simulink model "trimming_find_initial_value"  (R2022a)
settings: Solver=VariableStepAuto  StartTime=0.0  StopTime=0.1  RelTol=1e-3
values from neighbouring files (symbols this model uses):
  h = xMax-xMin    [LP_BasicSolution.m]    (also in LP_def.m = [uMax-up; LP_lift.m = [uMax-up; LP_sig.m = [uMax-up; LP_thrust.m = [uMax-up)
  m = m1-1    [CGIwrap.m]    (also in DAISY_CHAINING.m; DA_Allocation.m; LP_BasicSolution.m; LP_def.m)
undefined symbols (not defined in the file or in its folder): ft, kg, km, s, slug
libraries: aerolibconvert2 x12, sharedtransform x2, aerolibatmos2 x1
settings Model: Creator=user
settings SolverCC: AlgebraicLoopSolver=TrustRegion
settings DebuggingCC: UnconnectedInputMsg=warning  UnconnectedOutputMsg=warning  UnconnectedLineMsg=warning  SFMachineParentedDataDiag=warning

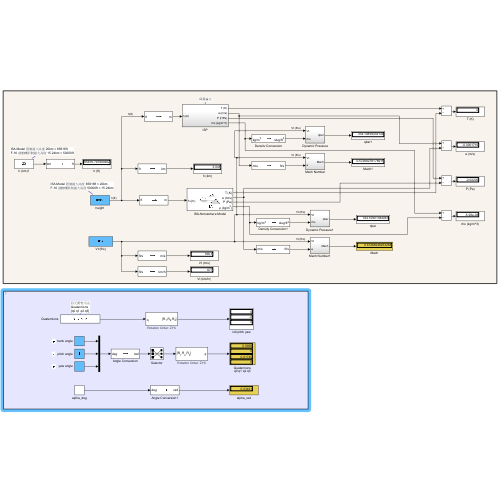
[thumbnail: Simulink's stored preview of the top-level diagram]
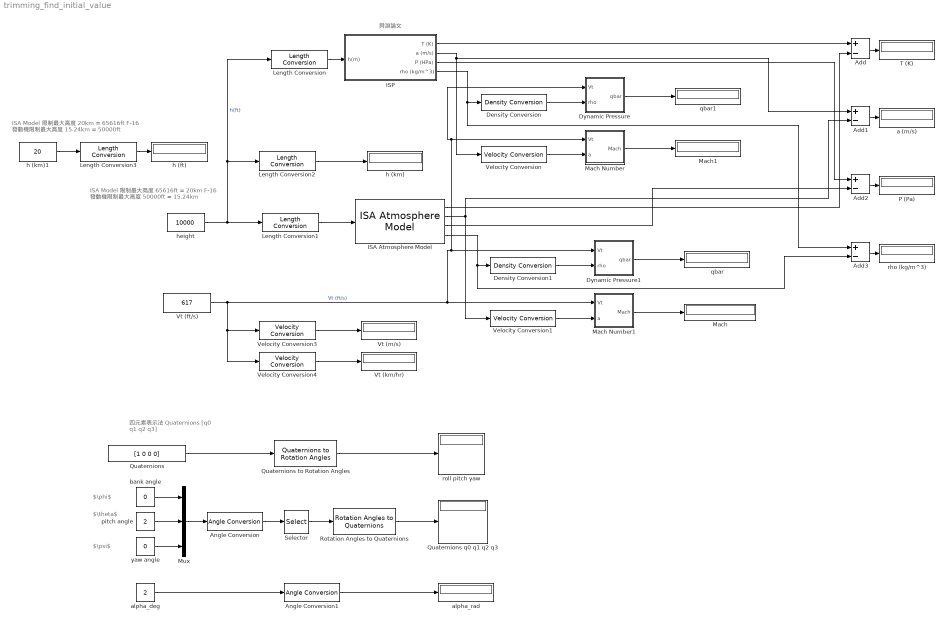
== system trimming_find_initial_value ==
  note: $\phi$
  note: 舜淵論文
  note: ISA Model 限制最大高度 65616ft = 20km
      | F-16 發動機限制最大高度 50000ft = 15.24km
  note: ISA Model 限制最大高度 20km = 65616ft
      | F-16 發動機限制最大高度 15.24km = 50000ft
  note: 四元素表示法
      | Quaternions
      | [q0 q1 q2 q3]
  note: $\theta$
  note: $\psi$
  Add{,1..3} (4 alike) : Sum  Inputs=+-
  Angle Conversion : aerolibconvert2/Angle Conversion  IU=deg  OU=rad
  Angle Conversion1 : aerolibconvert2/Angle Conversion  IU=deg  OU=rad
  Density Conversion : aerolibconvert2/Density Conversion  IU=kg/m^3  OU=slug/ft^3
      settings: SourceProductBaseCode=AE
  Density Conversion1 : aerolibconvert2/Density Conversion  IU=kg/m^3  OU=slug/ft^3
      settings: SourceProductBaseCode=AE
  Dynamic Pressure : Subsystem
  Dynamic Pressure1 : Subsystem
  ISA Atmosphere Model : aerolibatmos2/ISA Atmosphere Model  custom=off  g=9.80665  gamma=1.4  R=287.0531  L=0.0065  h_trop=11000  h_strat=20000  rho0=1.225  P0=101325  T0=288.15  h0=0
  "ISP " : Subsystem
  Length Conversion : aerolibconvert2/Length Conversion  IU=ft  OU=m
  Length Conversion1 : aerolibconvert2/Length Conversion  IU=ft  OU=m
  Length Conversion2 : aerolibconvert2/Length Conversion  IU=ft  OU=km
  Length Conversion3 : aerolibconvert2/Length Conversion  IU=km  OU=ft
  Mach : Display
  Mach Number : Subsystem
  Mach Number1 : Subsystem
  Mach1 : Display
  Mux : Mux  Inputs=3
  P (Pa) : Display
  Quaternions : Constant  Value=[1 0 0 0]
  Quaternions q0 q1 q2 q3 : Display
  Quaternions to Rotation Angles : sharedtransform/Quaternions to Rotation Angles  rotationOrder=ZYX  aMode=aMode
      settings: SourceProductBaseCode=AE,PW,DR,MT,VE
  Rotation Angles to Quaternions : sharedtransform/Rotation Angles to Quaternions  rotationOrder=ZYX  aMode=aMode
      settings: SourceProductBaseCode=AE,PW,DR,MT,VE
  Selector : Selector  InputPortWidth=3  IndexOptions=Index vector (dialog)  Indices=[3 2 1]  OutputSizes=1
  T (K) : Display
  Velocity Conversion : aerolibconvert2/Velocity Conversion  IU=m/s  OU=ft/s
  Velocity Conversion1 : aerolibconvert2/Velocity Conversion  IU=m/s  OU=ft/s
  Velocity Conversion3 : aerolibconvert2/Velocity Conversion  IU=ft/s  OU=m/s
  Velocity Conversion4 : aerolibconvert2/Velocity Conversion  IU=ft/s  OU=km/h
  Vt (ft/s) : Constant  Value=617
  Vt (km/hr) : Display
  Vt (m/s) : Display
  a (m/s) : Display
  alpha_deg : Constant  Value=2
  alpha_rad : Display
  bank angle : Constant  Value=0
  h (ft) : Display
  h (km) : Display
  h (km)1 : Constant  Value=20
  height : Constant  Value=10000
  pitch angle : Constant  Value=2
  qbar : Display
  qbar1 : Display
  rho (kg/m^3) : Display
  roll pitch yaw : Display
  yaw angle : Constant  Value=0
  wires:
  "ISP "/4(rho (kg/m^3)) -> Add3/1, Density Conversion/1
  "ISP "/3(P (HPa)) -> Add2/1
  "ISP "/2(a (m/s)) -> Add1/1, Velocity Conversion/1
  Dynamic Pressure/1(qbar) -> qbar1/1
  Mach Number/1(Mach) -> Mach1/1
  Density Conversion/1 -> Dynamic Pressure/2(rho)
  height/1 -> Length Conversion2/1, Length Conversion/1, Length Conversion1/1  "h(ft)"
  Length Conversion/1 -> "ISP "/1(h(m))
  Vt (ft/s)/1 -> Velocity Conversion4/1, Velocity Conversion3/1, Dynamic Pressure/1(Vt), Mach Number/1(Vt), Dynamic Pressure1/1(Vt), Mach Number1/1(Vt)  "Vt (ft/s)"
  Velocity Conversion/1 -> Mach Number/2(a)
  "ISP "/1(T (K)) -> Add/1
  Velocity Conversion1/1 -> Mach Number1/2(a)
  Length Conversion1/1 -> ISA Atmosphere Model/1
  ISA Atmosphere Model/3 -> Add2/2
  ISA Atmosphere Model/4 -> Add3/2, Density Conversion1/1
  Density Conversion1/1 -> Dynamic Pressure1/2(rho)
  ISA Atmosphere Model/1 -> Add/2
  ISA Atmosphere Model/2 -> Add1/2, Velocity Conversion1/1
  Dynamic Pressure1/1(qbar) -> qbar/1
  Mach Number1/1(Mach) -> Mach/1
  Add/1 -> T (K)/1
  Add1/1 -> a (m/s)/1
  Add2/1 -> P (Pa)/1
  Add3/1 -> rho (kg/m^3)/1
  Length Conversion2/1 -> h (km)/1
  Velocity Conversion3/1 -> Vt (m/s)/1
  Velocity Conversion4/1 -> Vt (km/hr)/1
  Length Conversion3/1 -> h (ft)/1
  h (km)1/1 -> Length Conversion3/1
  Angle Conversion1/1 -> alpha_rad/1
  Angle Conversion/1 -> Selector/1
  Mux/1 -> Angle Conversion/1
  pitch angle/1 -> Mux/2
  bank angle/1 -> Mux/1
  yaw angle/1 -> Mux/3
  alpha_deg/1 -> Angle Conversion1/1
  Rotation Angles to Quaternions/1 -> Quaternions q0 q1 q2 q3/1
  Selector/1 -> Rotation Angles to Quaternions/1
  Quaternions to Rotation Angles/1 -> roll pitch yaw/1
  Quaternions/1 -> Quaternions to Rotation Angles/1

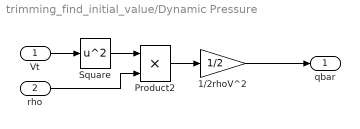
== system trimming_find_initial_value/Dynamic Pressure ==
  Vt : Inport
  rho : Inport  Port=2
  1/2rhoV^2 : Gain  Gain=1/2  SaturateOnIntegerOverflow=on  OutDataTypeStr=Inherit: Same as input  ParamDataTypeStr=Inherit: Same as input
  Product2 : Product  InputSameDT=on  SaturateOnIntegerOverflow=on  OutDataTypeStr=Inherit: Same as first input
  Square : Math  Operator=square  SignedPower=on
  qbar : Outport
  wires:
  rho/1 -> Product2/2
  Square/1 -> Product2/1
  1/2rhoV^2/1 -> qbar/1
  Product2/1 -> 1/2rhoV^2/1
  Vt/1 -> Square/1

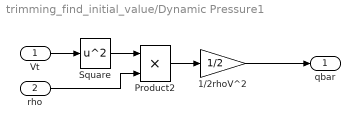
== system trimming_find_initial_value/Dynamic Pressure1 ==
  Vt : Inport
  rho : Inport  Port=2
  1/2rhoV^2 : Gain  Gain=1/2  SaturateOnIntegerOverflow=on  OutDataTypeStr=Inherit: Same as input  ParamDataTypeStr=Inherit: Same as input
  Product2 : Product  InputSameDT=on  SaturateOnIntegerOverflow=on  OutDataTypeStr=Inherit: Same as first input
  Square : Math  Operator=square  SignedPower=on
  qbar : Outport
  wires:
  rho/1 -> Product2/2
  Square/1 -> Product2/1
  1/2rhoV^2/1 -> qbar/1
  Product2/1 -> 1/2rhoV^2/1
  Vt/1 -> Square/1

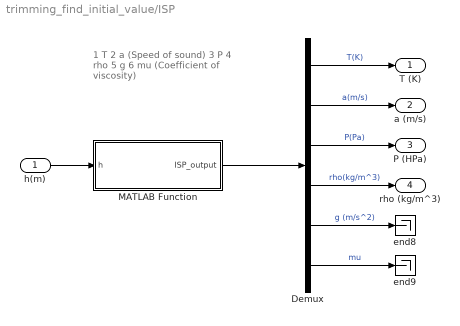
== system trimming_find_initial_value/ISP  ==
  note: 1 T
      | 2 a (Speed of sound)
      | 3 P
      | 4 rho
      | 5 g
      | 6 mu (Coefficient of viscosity)
  h(m) : Inport
  Demux : Demux  Outputs=[1,1,1,1,1,1]
      settings: DisplayOption=none
  MATLAB Function : MATLAB Function  TreatAsAtomicUnit=on
  end8 : Terminator
  end9 : Terminator
  T (K) : Outport  VectorParamsAs1DForOutWhenUnconnected=off
  a (m/s) : Outport  Port=2  VectorParamsAs1DForOutWhenUnconnected=off
  P (HPa) : Outport  Port=3  VectorParamsAs1DForOutWhenUnconnected=off
  rho (kg/m^3) : Outport  Port=4  VectorParamsAs1DForOutWhenUnconnected=off
  wires:
  MATLAB Function/1(ISP_output) -> Demux/1
  h(m)/1 -> MATLAB Function/1(h)
  Demux/4 -> rho (kg/m^3)/1  "rho(kg/m^3)"
  Demux/2 -> a (m/s)/1  "a(m/s)"
  Demux/1 -> T (K)/1  "T(K)"
  Demux/5 -> end8/1  "g (m/s^2)"
  Demux/6 -> end9/1  "mu"
  Demux/3 -> P (HPa)/1  "P(Pa)"

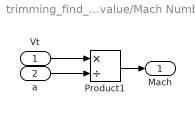
== system trimming_find_initial_value/Mach Number ==
  Vt : Inport
  a : Inport  Port=2
  Product1 : Product  Inputs=*/  InputSameDT=on  SaturateOnIntegerOverflow=on  OutDataTypeStr=Inherit: Same as first input
  Mach : Outport  Unit=1  VectorParamsAs1DForOutWhenUnconnected=off
  wires:
  Vt/1 -> Product1/1
  a/1 -> Product1/2
  Product1/1 -> Mach/1

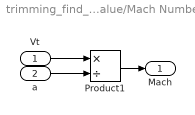
== system trimming_find_initial_value/Mach Number1 ==
  Vt : Inport
  a : Inport  Port=2
  Product1 : Product  Inputs=*/  InputSameDT=on  SaturateOnIntegerOverflow=on  OutDataTypeStr=Inherit: Same as first input
  Mach : Outport  Unit=1  VectorParamsAs1DForOutWhenUnconnected=off
  wires:
  Vt/1 -> Product1/1
  a/1 -> Product1/2
  Product1/1 -> Mach/1

== matlab function trimming_find_initial_value/ISP /MATLAB Function ==
  data: h input; ISP_output output
function ISP_output =ISP(h)
%%  Symbol:
% a = Speed of sound.
% C = The temperature in Celsius.
% Cv = Constant volime ; Cv = e(internal energy)/T.
% Cp = Constant pressure ; Cp = h(enthalpy)/T.
% e = Internal energy.
% e_tr = Translational energy.
% e_rot = Rotational energy.
% e_vib = Vibrational energy.
% g = Is the gravitational acceleration at height h above sea level.
% go = Is the standard gravitational acceleration.
% gamma = Define Cp(constant pressure)/Cv(constant volime).
% h = Geometric altitude.
% mu = Coefficient of viscosity.
% P = The standard atmosphere at h.
% re = Is the Earth's mean radius.
% R = The gas constant for air.
% T = Is temperature in K.
% To = Is the sea_level temperature (absolute).
% rho = Density.
%% Gravitational acceleration 
go=9.806645;     % m/s^2
re=6356766;      % m
g=go*(re/(re+h))^2;
%%  Standard Atmosphere and Temperature
if h<11000 %11000m 以下
    P = (1013.25*(1-(2.25577e-5*h))^5.255879)*100 ;%unit Pa
    T = 288.15-((6.5e-3*h)); %unit K
elseif h ==11000
    P = 2.263203776117090e+04; %unit Pa
    T = 216.6500; %unit K
elseif h>11000 && h<20000 
    P = (226.32*exp(-0.000157688*(h-11000)) )*100; %unit Pa
    T = 216.6500; %unit K
elseif h==20000
    P = 5.474893557709153e+03; %unit Pa
    T = 216.6500; %unit K
else
    P = (54.7482*((1+4.61574e-6*(h-20000)))^-34.163215)*100 ; %unit Pa
    T = 216.6500+1e-3*(h-20000);%unit K
end
%%  Density
% The gas constant for air in SI units [(N*m)/(kg*K)].
R=287.0528;
rho=P/(R*T);
%%  Coefficient of viscosity
% Viscosity in SI units [kg/(s*m)].
mu=1.458*(10^-6)*((T^1.5)/(T+110.4));
%%  Speed of sound 
% molecular energy.
e_tr=(3/2)*R*T;
e_rot=R*T;
e_vib=(1/2)*R*T;
if ( T >= 600 ) % when the air temperature reaches 600K or higher .
    e=e_tr+e_rot+e_vib;
    Cv=e/T;
    Cp=(e+R*T)/T;
else
    e=e_tr+e_rot;
    Cv=e/T;
    Cp=(e+R*T)/T;
end
gamma=Cp/Cv;
% Speed of sound .
a=sqrt(gamma*R*T);
%%
ISP_output = [T,a,P,rho,g,mu];
